simulink model "Isolated_buck"  (R2023b)
settings: Solver=VariableStepAuto  StartTime=0.0  StopTime=10  RelTol=1e-3
libraries: spsVoltageMeasurementLib x4, spsIGBTLib x4, spsSeriesRLCBranchLib x3, spsDiodeLib x2, spsDCVoltageSourceLib x1, spsLinearTransformerLib x1, eeGeneralControl x1, spsTriangleGeneratorLib x1, sps_lib x1
settings Model: NumberOfSteps=10  Creator=Admin  LastModifiedBy=Admin

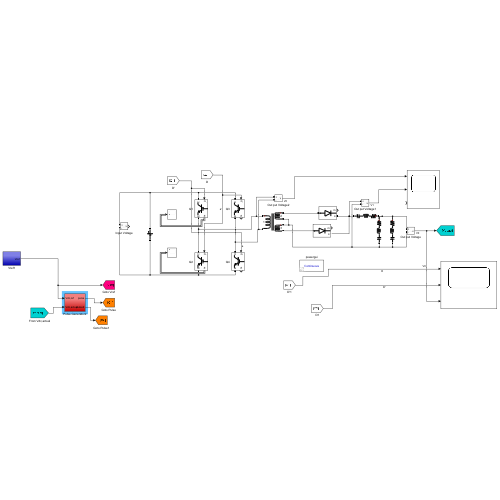
[thumbnail: Simulink's stored preview of the top-level diagram]
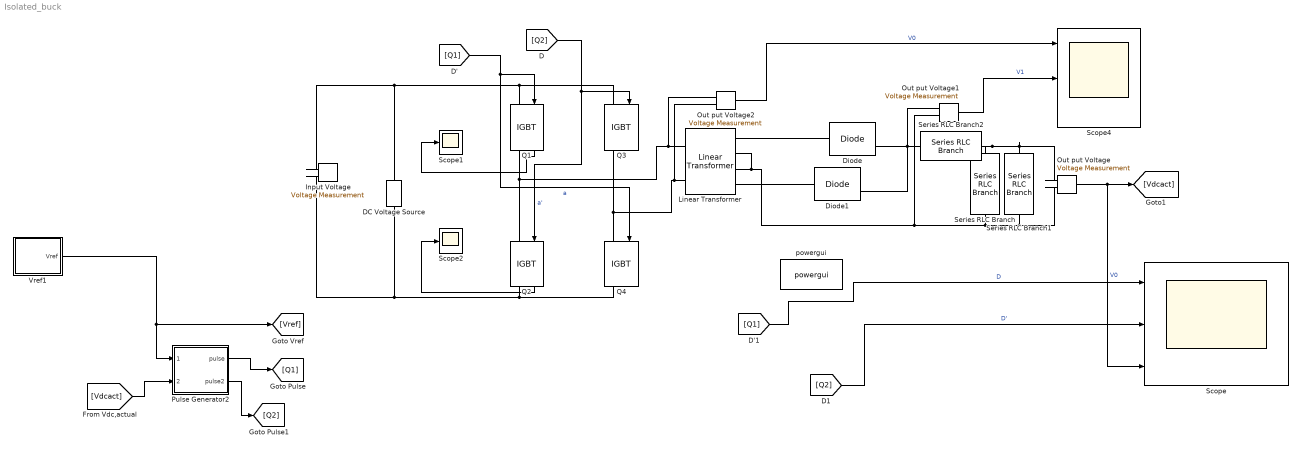
== system Isolated_buck ==
  DC Voltage Source : spsDCVoltageSourceLib/DC Voltage Source  Amplitude=400  Measurements=None
  Diode : spsDiodeLib/Diode  Ron=0  Lon=0  Vf=0  IC=0  UseSnubber=0  Rs=0  Cs=0  Measurements=on
  Diode1 : spsDiodeLib/Diode  Ron=0  Lon=0  Vf=0  IC=0  UseSnubber=0  Rs=0  Cs=0  Measurements=on
  Input Voltage : spsVoltageMeasurementLib/Voltage Measurement  PhasorSimulation=off  OutputType=Complex  PSBequivalent=0
  Linear Transformer : spsLinearTransformerLib/Linear Transformer  UNITS=SI  NominalPower=[ 1000 50 ]  winding1=[400 1e-3 0]  winding2=[200 1e-3 0]  ThreeWindings=on  winding3=[200 1e-3 0 ]  RmLm=[1e-3 50e-3]  Measurements=Magnetization current  DataType=on
  Out put Voltage : spsVoltageMeasurementLib/Voltage Measurement  PhasorSimulation=off  OutputType=Complex  PSBequivalent=0
  Out put Voltage1 : spsVoltageMeasurementLib/Voltage Measurement  PhasorSimulation=off  OutputType=Complex  PSBequivalent=0
  Out put Voltage2 : spsVoltageMeasurementLib/Voltage Measurement  PhasorSimulation=off  OutputType=Complex  PSBequivalent=0
  Pulse Generator2 : Subsystem
  Q{1..4} (4 alike) : spsIGBTLib/IGBT  Ron=0  Lon=0  Vf=0  Tf=1e-6  Tt=2e-6  IC=0  Rs=0  Cs=0  Measurements=on
  Scope : Scope  NumInputPorts=3
  Scope1 : Scope
  Scope2 : Scope
  Scope4 : Scope  NumInputPorts=3
  Series RLC Branch : spsSeriesRLCBranchLib/Series RLC Branch  LConnTagsString=__new0  RConnTagsString=__new0  BranchType=RLC  Resistance=1e-9  Inductance=0  SetiL0=off  InitialCurrent=0  Capacitance=13.54e-6  Setx0=off  InitialVoltage=0  Measurements=None
  Series RLC Branch1 : spsSeriesRLCBranchLib/Series RLC Branch  LConnTagsString=__new0  RConnTagsString=__new0  BranchType=RLC  Resistance=2.304  Inductance=0  SetiL0=off  InitialCurrent=0  Capacitance=0  Setx0=off  InitialVoltage=0  Measurements=None
  Series RLC Branch2 : spsSeriesRLCBranchLib/Series RLC Branch  LConnTagsString=__new0  RConnTagsString=__new0  BranchType=RLC  Resistance=1e-9  Inductance=1.2e-3  SetiL0=off  InitialCurrent=0  Capacitance=0  Setx0=off  InitialVoltage=0  Measurements=None
  Vref1 : Subsystem
  powergui : sps_lib/powergui  Priority=1  SimulationMode=Continuous  SampleTime=50e-6  frequency=60  Iterations=50  frequencyindice=0  Pbase=100e6  ErrMax=1e-4  UnitsV=kV  UnitsW=MW  buscounter=0  FunctionMessages=off  echomessages=off  EnableUseOfTLC=off  CurrentSourceSwitches=off  DisableSnubberDevices=off  DisableRonSwitches=off  DisableVfSwitches=off  DisplayEquations=off  AutomaticDiscreteSolvers=off  SolverType=Tustin/Backward Euler (TBE)  Interpol=off  ExternalGateDelay=off  methode=off  Ts=100  x0status=blocks  SPID=on  SwTol=0  HookPort=off  NonlinearTolerance=1e-4  nMaxIteration=100  ContinueOnMaxIteration=off  RestoreLinks=warning  ResistiveCurrentMeasurement=off  Frange=[0:2:500]  Ylog=off  Xlog=on  ShowGrid=off  save=off  variable=ZData  structure=0  ZoomFFT=off  StartTime=0.0  cycles=1  DisplayStyle=1  fundamental=60  FreqAxis=off  MaxFrequency=1000  frequencyindicesteady=1  RmsSteady=1  display=off
  wires:
  [Q1] -> Q4/1, Q1/1  "a"
  [Q2] -> Q2/1, Q3/1  "a'"
  Out put Voltage/1 -> [Vdcact], Scope/3  "V0"
  [Q2] -> Scope/2  "D'"
  [Q1] -> Scope/1  "D"
  Q1/1 -> Scope1/1
  Q2/1 -> Scope2/1
  Out put Voltage2/1 -> Scope4/1  "V0"
  Out put Voltage1/1 -> Scope4/2  "V1"
  [Vdcact] -> Pulse Generator2/2(Vdc,actual)
  Pulse Generator2/1(pulse) -> [Q1]
  Pulse Generator2/2(pulse2) -> [Q2]
  Vref1/1(Vref) -> [Vref], Pulse Generator2/1(Vdc,ref)
  connections:
  Q1/LConn1 -- DC Voltage Source/RConn1 -- Input Voltage/LConn1 -- Q3/LConn1
  Q4/RConn1 -- Input Voltage/LConn2 -- DC Voltage Source/LConn1 -- Q2/RConn1
  Out put Voltage/LConn1 -- Series RLC Branch1/LConn1 -- Series RLC Branch/LConn1 -- Series RLC Branch2/LConn1
  Linear Transformer/RConn1 -- Diode/LConn1
  Series RLC Branch1/RConn1 -- Out put Voltage/LConn2 -- Out put Voltage1/LConn2 -- Linear Transformer/RConn3 -- Linear Transformer/RConn2 -- Series RLC Branch/RConn1
  Out put Voltage2/LConn2 -- Q3/RConn1 -- Q4/LConn1 -- Linear Transformer/LConn2
  Q1/RConn1 -- Out put Voltage2/LConn1 -- Linear Transformer/LConn1 -- Q2/LConn1
  Diode1/RConn1 -- Diode/RConn1 -- Out put Voltage1/LConn1 -- Series RLC Branch2/RConn1
  Linear Transformer/RConn4 -- Diode1/LConn1

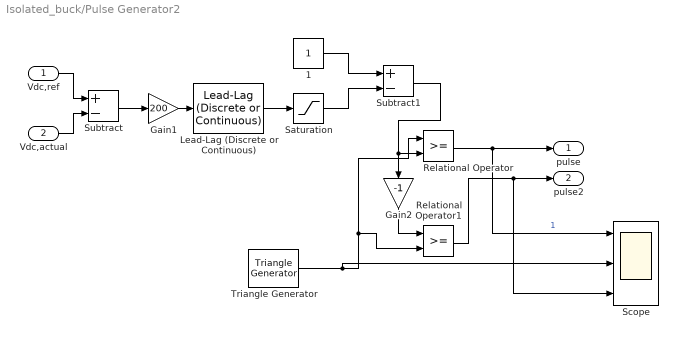
== system Isolated_buck/Pulse Generator2 ==
  Vdc,ref : Inport
  Vdc,actual : Inport  Port=2
  1 : Constant
  Gain1 : Gain  Gain=200
  Gain2 : Gain  Gain=-1
  Lead-Lag (Discrete or Continuous) : eeGeneralControl/Lead-Lag (Discrete or Continuous)  T1=1  T2=10  B=inf  A=-inf  init_option=Specify as parameter  x0=0  Ts=-1
      settings: LibrarySourceBlock=|
      | ee_sl_lib/General Control/Lead-Lag
      | (Discrete or Continuous)
  Relational Operator : RelationalOperator  OutDataTypeStr=boolean  RndMeth=Simplest  InputSameDT=off
  Relational Operator1 : RelationalOperator  OutDataTypeStr=boolean  RndMeth=Simplest  InputSameDT=off
  Saturation : Saturate  UpperLimit=1  LowerLimit=-1
  Scope : Scope  NumInputPorts=3
  Subtract : Sum  Inputs=+-
  Subtract1 : Sum  Inputs=+-
  Triangle Generator : spsTriangleGeneratorLib/Triangle Generator  Freq=10e3  Phase=90  Ts=0
  pulse : Outport
  pulse2 : Outport  Port=2
  wires:
  Subtract/1 -> Gain1/1
  Lead-Lag (Discrete or Continuous)/1 -> Saturation/1
  Saturation/1 -> Subtract1/2
  Vdc,actual/1 -> Subtract/2
  Vdc,ref/1 -> Subtract/1
  Relational Operator1/1 -> Scope/3, pulse2/1
  Relational Operator/1 -> Scope/1, pulse/1  "1"
  Triangle Generator/1 -> Scope/2, Relational Operator/1, Relational Operator1/2
  Gain2/1 -> Relational Operator1/1
  Gain1/1 -> Lead-Lag (Discrete or Continuous)/1
  1/1 -> Subtract1/1
  Subtract1/1 -> Gain2/1, Relational Operator/2

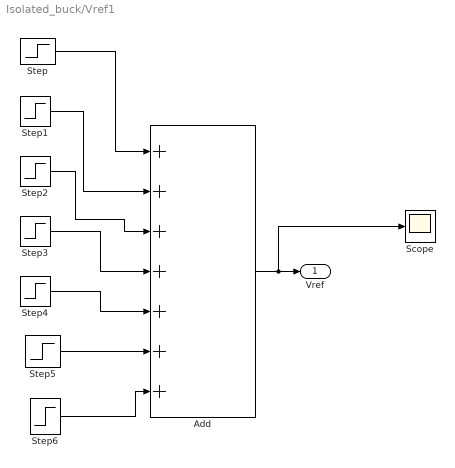
== system Isolated_buck/Vref1 ==
  Add : Sum  Inputs=+++++++
  Scope : Scope
  Step : Step  Time=0.1  Before=40  After=80  SampleTime=0
  Step1 : Step  Time=0.1  After=-50  SampleTime=0
  Step2 : Step  Time=0.2  After=10  SampleTime=0
  Step3 : Step  Time=0.4  After=10  SampleTime=0
  Step4 : Step  Time=0.1  After=10  SampleTime=0
  Step5 : Step  Time=0.1  After=10  SampleTime=0
  Step6 : Step  Time=0.1  After=10  SampleTime=0
  Vref : Outport
  wires:
  Add/1 -> Scope/1, Vref/1
  Step6/1 -> Add/7
  Step5/1 -> Add/6
  Step4/1 -> Add/5
  Step3/1 -> Add/4
  Step2/1 -> Add/3
  Step1/1 -> Add/2
  Step/1 -> Add/1
